simulink model "vrsvdex"  (Simulink 3.00)
settings: Solver=FixedStepDiscrete  StartTime=0.0  StopTime=499  RelTol=1e-3
undefined symbols (not defined in the file or in its folder): m, n
libraries: smxl x8, simulink3 x1
settings Model: LastModifiedBy=giampiero

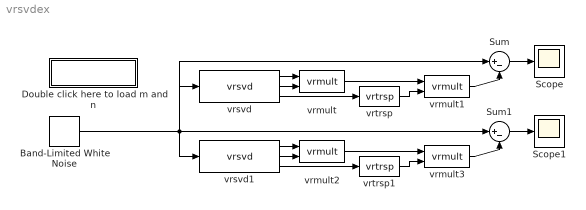
== system vrsvdex ==
  Band-Limited White Noise : simulink3/Sources/Band-Limited White Noise  Cov=[0.1]*ones(n*m,1)  Ts=0.1  seed=1:(n*m)
  "Double click here to load m and n " : Subsystem
      settings: OpenFcn=m=2;n=3;
      mask Display: disp('Load m and n')
  Scope : Scope
      settings: TimeRange=500  YMin=-1e-014  YMax=1e-014  SaveToWorkspace=off  SaveName=ScopeData
  Scope1 : Scope
      settings: TimeRange=500  YMin=-1e-014  YMax=1e-014  SaveToWorkspace=off  SaveName=ScopeData
  Sum : Sum  Inputs=|+-  SaturateOnIntegerOverflow=on
  Sum1 : Sum  Inputs=|+-  SaturateOnIntegerOverflow=on
  vrmult : smxl/Real Matrices/vrmult  dims=[n min(m,n) min(m,n)]
  vrmult1 : smxl/Real Matrices/vrmult  dims=[n min(m,n) m]
  vrmult2 : smxl/Real Matrices/vrmult  dims=[m min(m,n) min(m,n)]
  vrmult3 : smxl/Real Matrices/vrmult  dims=[m min(m,n) n]
  vrsvd : smxl/Real Matrices/vrsvd  dims=[n m]
  vrsvd1 : smxl/Real Matrices/vrsvd  dims=[m n]
  vrtrsp : smxl/Real Matrices/vrtrsp  dims=[m min(m,n)]
  vrtrsp1 : smxl/Real Matrices/vrtrsp  dims=[n min(m,n)]
  wires:
  vrmult1/1 -> Sum/2
  Band-Limited White Noise/1 -> vrsvd/1, Sum/1, vrsvd1/1, Sum1/1
  Sum/1 -> Scope/1
  vrsvd1/1 -> vrmult2/1
  vrmult2/1 -> vrmult3/1
  vrmult3/1 -> Sum1/2
  Sum1/1 -> Scope1/1
  vrsvd1/3 -> vrtrsp1/1
  vrsvd1/2 -> vrmult2/2
  vrtrsp1/1 -> vrmult3/2
  vrsvd/1 -> vrmult/1
  vrsvd/2 -> vrmult/2
  vrsvd/3 -> vrtrsp/1
  vrmult/1 -> vrmult1/1
  vrtrsp/1 -> vrmult1/2

== system vrsvdex/Double click here to load m and n  ==
